simulink model "a1__MoHinh"  (R2019a)
settings: Solver=VariableStepAuto  StartTime=0.0  StopTime=8  RelTol=1e-3
libraries: commsynccomp2 x1, dsparch4 x1, dspsigops x1
settings Model: Creator=Thanh_Hai  LastModifiedBy=Thanh_Hai

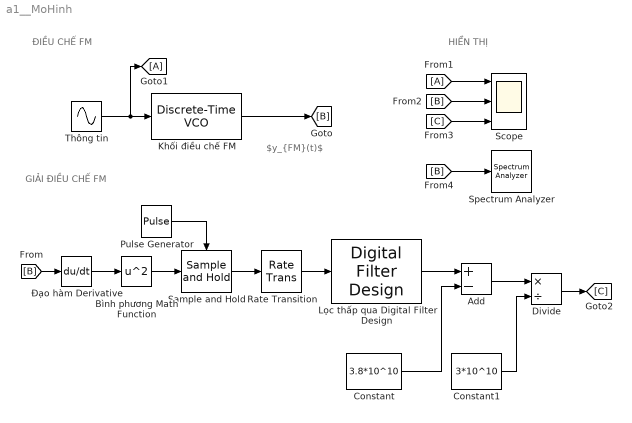
== system a1__MoHinh ==
  note: HIỂN THỊ
  note: GIẢI ĐIỀU CHẾ FM
  note: ĐIỀU CHẾ FM
  note: $y_{FM}(t)$
  Add : Sum  Inputs=+-
  Bình phương Math Function : Math  Operator=square  SaturateOnIntegerOverflow=on
  Constant : Constant  Value=3.8*10^10
  Constant1 : Constant  Value=3*10^10
  Divide : Product  Inputs=*/
  "Khối điều chế FM " : commsynccomp2/Discrete-Time VCO  Ac=5  Fc=3000  Kc=2000  Ph=0  ts=1/20000
      settings: SourceProductName=Communications Toolbox  SourceProductBaseCode=CM
  Lọc thấp qua Digital Filter Design : dsparch4/Digital Filter Design  mwdsp_browser_bugfix_var=off
  Pulse Generator : DiscretePulseGenerator  PulseType=Time based  Period=1/40000  PulseWidth=50
  Rate Transition : RateTransition  OutPortSampleTime=1/40000
  Sample and Hold : dspsigops/Sample and Hold  trig=Rising edge  initCond=0  latchinput=off
  Scope : Scope  NumInputPorts=3
  Spectrum Analyzer : SpectrumAnalyzer
  "Thông tin " : Sin  Frequency=2*pi*500  SampleTime=1/20000
  Đạo hàm Derivative : Derivative
  wires:
  "Thông tin "/1 -> "Khối điều chế FM "/1, [A]
  [A] -> Scope/1
  "Khối điều chế FM "/1 -> [B]
  Đạo hàm Derivative/1 -> Bình phương Math Function/1
  [B] -> Đạo hàm Derivative/1
  Constant/1 -> Add/2
  Bình phương Math Function/1 -> Sample and Hold/1
  Pulse Generator/1 -> Sample and Hold/Trigger
  Sample and Hold/1 -> Rate Transition/1
  Rate Transition/1 -> Lọc thấp qua Digital Filter Design/1
  Lọc thấp qua Digital Filter Design/1 -> Add/1
  Add/1 -> Divide/1
  [B] -> Scope/2
  [C] -> Scope/3
  Constant1/1 -> Divide/2
  [B] -> Spectrum Analyzer/1
  Divide/1 -> [C]
